simulink model "Magnetorquer_Model"  (R2024a)
settings: Solver=VariableStepAuto  StartTime=0.0  StopTime=10.0  RelTol=1e-3
settings Model: Creator=hendr  LastModifiedBy=hendr

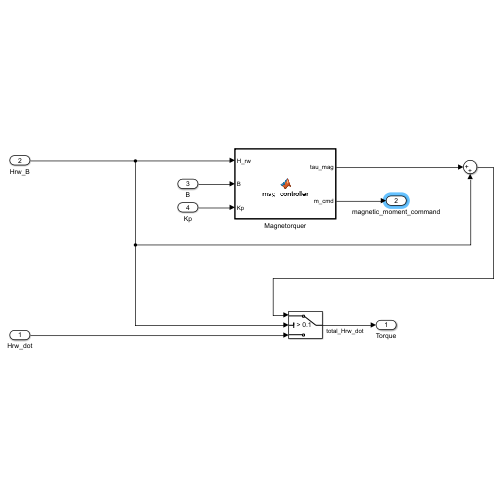
[thumbnail: Simulink's stored preview of the top-level diagram]
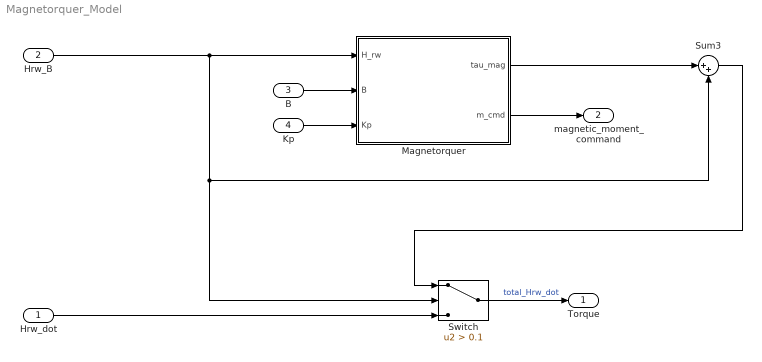
== system Magnetorquer_Model ==
  Hrw_dot : Inport
  Hrw_B : Inport  Port=2
  B : Inport  Port=3
  Kp : Inport  Port=4
  Magnetorquer : MATLAB Function  TreatAsAtomicUnit=on
  Sum3 : Sum  Inputs=|++
  Switch : Switch  Criteria=u2 > Threshold  Threshold=0.1  SaturateOnIntegerOverflow=off  InputSameDT=off
  Torque : Outport
  magnetic_moment_command : Outport  Port=2
  wires:
  Hrw_B/1 -> Switch/2, Sum3/2, Magnetorquer/1(H_rw)
  B/1 -> Magnetorquer/2(B)
  Kp/1 -> Magnetorquer/3(Kp)
  Hrw_dot/1 -> Switch/3
  Magnetorquer/2(m_cmd) -> magnetic_moment_command/1
  Magnetorquer/1(tau_mag) -> Sum3/1
  Sum3/1 -> Switch/1
  Switch/1 -> Torque/1  "total_Hrw_dot"

== matlab function Magnetorquer_Model/Magnetorquer ==
  data: H_rw input; tau_mag output; B input; Kp input; m_cmd output
function [tau_mag, m_cmd] = mag_controller(H_rw, B, Kp)
    if norm(B) < 1e-9
        m_cmd = zeros(3,1); tau_mag = zeros(3,1); return;
    end
    tau_des = -Kp * H_rw;                    % Desired unloading torque
    m_cmd = cross(tau_des, B) / (B'*B);      % Minimum norm solution
    m_cmd = saturate_moment(m_cmd, M_max);   % e.g. 20 A·m² per axis
    tau_mag = cross(m_cmd, B);
end
